simulink model "Disturbance_LQG_Stabilization_Simulink_Offline_Pendulum_Control"  (R2022b)
settings: Solver=VariableStepAuto  StartTime=0.0  StopTime=30  RelTol=1e-3
undefined symbols (not defined in the file or in its folder): A, A_kf, A_ob, B, B_kf, B_ob, C_full, C_kf, C_ob, D_full, D_kf, D_ob, K_lq, K_lq_alpha, Kpp, sigbuilder_block, voltage_max, x0
settings Model: Creator=utente  LastModifiedBy=federicocorso
settings SolverCC: AlgebraicLoopSolver=TrustRegion
settings DebuggingCC: UnconnectedInputMsg=warning  UnconnectedOutputMsg=warning  UnconnectedLineMsg=warning  SFMachineParentedDataDiag=warning
settings ModelReferenceCC: EnableRefExpFcnMdlSchedulingChecks=on

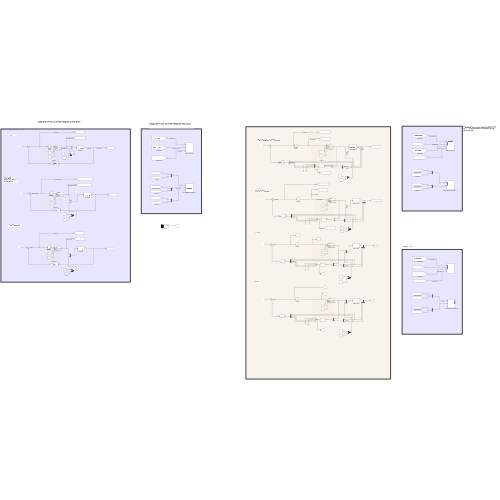
[thumbnail: Simulink's stored preview of the top-level diagram]
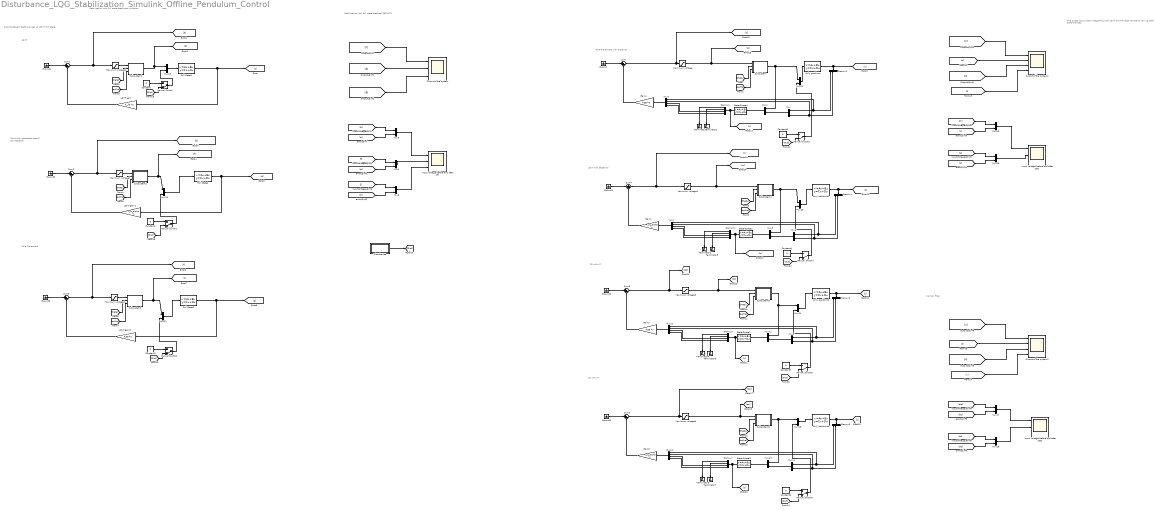
== system Disturbance_LQG_Stabilization_Simulink_Offline_Pendulum_Control ==
  note: LQ with KF
  note: PP with KF
  note: The closed loop system integrating both LQinf and PP observer seems having satisfactory performances.
  note: Kalman Filter
  note: Pole Placement with Observer
  note: Stabilization with full state feedback simulation
  note: LQinf
  note: Pole Placement Performances VS LQinf: Full State
  note: LQinf with prescribed rate of convergence
  note: Pole Placement
  note: Stabilization with full state feedback RESULTS
  note: LQinf with Observer
  Constant{,1..6} (7 alike) : Constant  Value=0
  Demux{1..8} (8 alike) : Demux
  Disturbance : Subsystem  Tag=STV Subsys  LoadFcn=sigbuilder_block('load',[516 294 550 400 ]);  StartFcn=sigbuilder_block('start');  StopFcn=sigbuilder_block('stop');  ClipboardFcn=sigbuilder_block('clipboard');  mask(Sigbuilder block){tuvar=[0:10]}
      mask help: Simulink:masks:SigbuilderBlock_MD
      mask init:
      | if ~strcmp(get_param(bdroot(gcbh),'SimulationStatus'),'stopped') tuvar = sigbuilder_block('maskInit'); end
      settings: CopyFcn=sigbuilder_block('copy');  DeleteFcn=sigbuilder_block('delete');  ModelCloseFcn=sigbuilder_block('modelClose');  PreSaveFcn=sigbuilder_block('preSave');  PauseFcn=sigbuilder_block('pause');  ContinueFcn=sigbuilder_block('continue');  NameChangeFcn=sigbuilder_block('namechange');  OpenFcn=sigbuilder_block('open',[516 294 550 400 ]);  CloseFcn=sigbuilder_block('close');
      mask Display: plot(0, 0, 100, 100,[2, 2, 32, 32, 2], [68, 8, 8, 68, 68],[32, 2], [38, 38], [32, 19, 2],[53, 60, 44], [32, 17, 17, 2],[16, 16, 31, 31]);txt = getActiveGroup(gcbh);text(2, 100, txt,'verticalAlignment', 'top');
  Full State1 : StateSpace  A=A  B=B  C=C_full  D=D_full  InitialCondition=x0
  Full State2 : StateSpace  A=A  B=B  C=C_full  D=D_full  InitialCondition=x0
  Full State3 : StateSpace  A=A  B=B  C=C_full  D=D_full  InitialCondition=x0
  Gain1 : Gain  Gain=K_lq_alpha  Multiplication=Matrix(K*u) (u vector)
  Gain2 : Gain  Gain=Kpp  Multiplication=Matrix(K*u) (u vector)
  Gain3 : Gain  Gain=K_lq_alpha  Multiplication=Matrix(K*u) (u vector)
  Gain4 : Gain  Gain=Kpp  Multiplication=Matrix(K*u) (u vector)
  Ground{,1..6} (7 alike) : Ground
  Input Voltage before and after sat : Scope  NumInputPorts=3
  Input Voltage before and after sat1 : Scope  NumInputPorts=3
  Input Voltage before and after sat2 : Scope  NumInputPorts=3
  LQinf gain : Gain  Gain=K_lq  Multiplication=Matrix(K*u) (u vector)
  LQinf gain1 : Gain  Gain=K_lq_alpha  Multiplication=Matrix(K*u) (u vector)
  LQinf gain2 : Gain  Gain=Kpp  Multiplication=Matrix(K*u) (u vector)
  Manual Switch{,1..6} (7 alike) : ManualSwitch  CurrentSetting=0
  Maximum voltage{,1..6} (7 alike) : Saturate  UpperLimit=voltage_max  LowerLimit=-voltage_max
  Mux{,2..6,8..9,11,13..25} (22 alike) : Mux  Inputs=2
  Mux{1,7,10,12} (4 alike) : Mux
  Only positions{,1..3} (4 alike) : StateSpace  A=A  B=B  C=C_full  D=D_full  InitialCondition=x0
  Output of the system : Scope  NumInputPorts=3
  Output of the system1 : Scope  NumInputPorts=4
  Output of the system2 : Scope  NumInputPorts=4
  State-Space1 : StateSpace  A=A_ob  B=B_ob  C=C_ob  D=D_ob  InitialCondition=[0;0;0;0]
  State-Space2 : StateSpace  A=A_kf  B=B_kf  C=C_kf  D=D_kf  InitialCondition=[0;0;0;0]
  State-Space3 : StateSpace  A=A_kf  B=B_kf  C=C_kf  D=D_kf  InitialCondition=[0;0;0;0]
  State-Space4 : StateSpace  A=A_ob  B=B_ob  C=C_ob  D=D_ob  InitialCondition=[0;0;0;0]
  Subsystem : Subsystem
  Subsystem1 : Subsystem
  Subsystem2 : Subsystem
  Subsystem3 : Subsystem
  Subsystem4 : Subsystem
  Subsystem5 : Subsystem
  Subsystem6 : Subsystem
  Sum{,1..6} (7 alike) : Sum  Inputs=|+-
  Terminator{,1..7} (8 alike) : Terminator
  wires:
  Maximum voltage/1 -> Subsystem/1(Control), [p]  "input Voltage PP"
  [theta] -> Subsystem/2(Theta)
  [aplha] -> Subsystem/3(Alpha)
  Ground/1 -> Sum/1
  Sum/1 -> [o], Maximum voltage/1  "erroro PP"
  Gain4/1 -> Sum/2
  Mux2/1 -> State-Space4/1  "Estimated States"
  State-Space4/1 -> [r], Demux1/1  "PP est"
  Subsystem/1(control) -> Mux2/1, Mux22/1
  Sum1/1 -> Maximum voltage1/1, [a]  "error LQinf"
  Ground1/1 -> Sum1/1
  Full State1/1 -> [c], LQinf gain/1  "Output LQinf"
  Subsystem1/1(control) -> [b], Mux19/1  "Input Voltage LQinf"
  Maximum voltage1/1 -> Subsystem1/1(Control)
  [aplha] -> Subsystem1/3(Alpha)
  [theta] -> Subsystem1/2(Theta)
  LQinf gain/1 -> Sum1/2
  Only positions/1 -> [n], Demux2/1  "Output PP"
  Mux/1 -> Mux2/2
  Demux2/2 -> Mux/2, Mux1/2  "alpha_sim"
  Demux2/1 -> Mux/1, Mux1/1  "theta_sim"
  Mux1/1 -> Gain4/1
  Demux1/3 -> Mux1/3
  Demux1/4 -> Mux1/4
  Demux1/1 -> Terminator/1
  Demux1/2 -> Terminator1/1
  [c] -> Output of the system/1  "Output LQinf"
  [b] -> Mux3/1
  [a] -> Mux3/2
  Mux3/1 -> Input Voltage before and after sat/1  "LQinf"
  Ground2/1 -> Sum2/1
  Full State2/1 -> [d], LQinf gain1/1  "Output LQinf_alpha"
  Sum2/1 -> Maximum voltage2/1, [e]  "error LQinf_alpha"
  Maximum voltage2/1 -> Subsystem2/1(Control)
  [aplha] -> Subsystem2/3(Alpha)
  LQinf gain1/1 -> Sum2/2
  Subsystem2/1(control) -> [f], Mux20/1  "Input Voltage LQinf_alpha"
  [theta] -> Subsystem2/2(Theta)
  [theta] -> Subsystem3/2(Theta)
  LQinf gain2/1 -> Sum3/2
  Sum3/1 -> Maximum voltage3/1, [h]  "error PP"
  Full State3/1 -> [g], LQinf gain2/1  "Output PP"
  Maximum voltage3/1 -> Subsystem3/1(Control)
  [aplha] -> Subsystem3/3(Alpha)
  Ground3/1 -> Sum3/1
  Subsystem3/1(control) -> [j], Mux21/1  "Input Voltage PP"
  [e] -> Mux4/2
  [f] -> Mux4/1
  Mux4/1 -> Input Voltage before and after sat/2  "LQinf_alpha"
  Mux5/1 -> Input Voltage before and after sat/3  "PP"
  [j] -> Mux5/1
  [h] -> Mux5/2
  [d] -> Output of the system/2  "Output LQinf_alpha"
  [g] -> Output of the system/3  "Output PP"
  Demux3/2 -> Terminator3/1
  Demux3/1 -> Terminator2/1
  Demux3/4 -> Mux7/4
  Demux3/3 -> Mux7/3
  Mux7/1 -> Gain1/1
  Demux4/1 -> Mux7/1, Mux6/1  "theta_sim"
  Demux4/2 -> Mux7/2, Mux6/2  "alpha_sim"
  Mux6/1 -> Mux8/2
  Only positions1/1 -> [k], Demux4/1  "Output LQinf"
  Subsystem4/1(control) -> Mux23/1, Mux8/1
  State-Space1/1 -> [q], Demux3/1  "LQinf est"
  Mux8/1 -> State-Space1/1  "Estimated States"
  Gain1/1 -> Sum4/2
  Sum4/1 -> Maximum voltage4/1, [l]  "error LQinf"
  Ground4/1 -> Sum4/1
  [aplha] -> Subsystem4/3(Alpha)
  [theta] -> Subsystem4/2(Theta)
  Maximum voltage4/1 -> Subsystem4/1(Control), [m]  "input Voltage LQinf"
  Maximum voltage5/1 -> [cc], Subsystem5/1(Control)
  [theta] -> Subsystem5/2(Theta)
  [aplha] -> Subsystem5/3(Alpha)
  Ground5/1 -> Sum5/1
  Sum5/1 -> [dd], Maximum voltage5/1  "not sat"
  Gain2/1 -> Sum5/2
  Mux11/1 -> State-Space2/1  "Estimated States"
  State-Space2/1 -> [v], Demux5/1
  Subsystem5/1(control) -> Mux24/1, Mux11/1
  Only positions2/1 -> [u], Demux6/1
  Mux9/1 -> Mux11/2
  Demux6/2 -> Mux9/2, Mux10/2  "alpha_sim"
  Demux6/1 -> Mux9/1, Mux10/1  "theta_sim"
  Mux10/1 -> Gain2/1
  Demux5/3 -> Mux10/3
  Demux5/4 -> Mux10/4
  Demux5/1 -> Terminator4/1
  Demux5/2 -> Terminator5/1
  Demux7/2 -> Terminator7/1
  Demux7/1 -> Terminator6/1
  Demux7/4 -> Mux12/4
  Demux7/3 -> Mux12/3
  Mux12/1 -> Gain3/1
  Demux8/1 -> Mux12/1, Mux14/1  "theta_sim"
  Demux8/2 -> Mux12/2, Mux14/2  "alpha_sim"
  Mux14/1 -> Mux13/2
  Only positions3/1 -> [s], Demux8/1
  Subsystem6/1(control) -> Mux25/1, Mux13/1
  State-Space3/1 -> [t], Demux7/1
  Mux13/1 -> State-Space3/1  "Estimated States"
  Gain3/1 -> Sum6/2
  Sum6/1 -> [bb], Maximum voltage6/1  "not sat"
  Ground6/1 -> Sum6/1
  [aplha] -> Subsystem6/3(Alpha)
  [theta] -> Subsystem6/2(Theta)
  Maximum voltage6/1 -> [aa], Subsystem6/1(Control)
  [n] -> Output of the system1/3  "Output PP sim"
  Mux16/1 -> Input Voltage before and after sat1/2  "PP"
  [p] -> Mux16/1
  [o] -> Mux16/2
  Mux15/1 -> Input Voltage before and after sat1/1  "LQinf"
  [l] -> Mux15/2
  [m] -> Mux15/1
  [k] -> Output of the system1/1  "Output LQinf sim"
  [q] -> Output of the system1/2  "Output LQinf est"
  [r] -> Output of the system1/4  "Output PP est"
  [v] -> Output of the system2/4  "Output PP est"
  [t] -> Output of the system2/2  "Output LQinf est"
  [s] -> Output of the system2/1  "Output LQinf sim"
  [aa] -> Mux17/1
  [bb] -> Mux17/2
  Mux17/1 -> Input Voltage before and after sat2/1  "LQinf"
  [dd] -> Mux18/2
  [cc] -> Mux18/1
  Mux18/1 -> Input Voltage before and after sat2/2  "PP"
  [u] -> Output of the system2/3  "Output PP sim"
  Mux19/1 -> Full State1/1
  Manual Switch/1 -> Mux19/2
  Manual Switch1/1 -> Mux20/2
  Manual Switch2/1 -> Mux21/2
  Manual Switch3/1 -> Mux22/2
  Manual Switch4/1 -> Mux23/2
  Manual Switch5/1 -> Mux24/2
  Mux24/1 -> Only positions2/1
  Mux23/1 -> Only positions1/1
  Mux22/1 -> Only positions/1
  Manual Switch6/1 -> Mux25/2
  Mux25/1 -> Only positions3/1
  Mux21/1 -> Full State3/1
  Mux20/1 -> Full State2/1
  [Dist] -> Manual Switch/2
  Constant/1 -> Manual Switch/1
  Constant2/1 -> Manual Switch2/1
  [Dist] -> Manual Switch2/2
  Constant1/1 -> Manual Switch1/1
  Constant3/1 -> Manual Switch3/1
  [Dist] -> Manual Switch3/2
  [Dist] -> Manual Switch4/2
  Constant4/1 -> Manual Switch4/1
  Constant5/1 -> Manual Switch5/1
  [Dist] -> Manual Switch5/2
  [Dist] -> Manual Switch6/2
  Constant6/1 -> Manual Switch6/1
  Disturbance/1(Signal 2) -> [Dist]
  [Dist] -> Manual Switch1/2

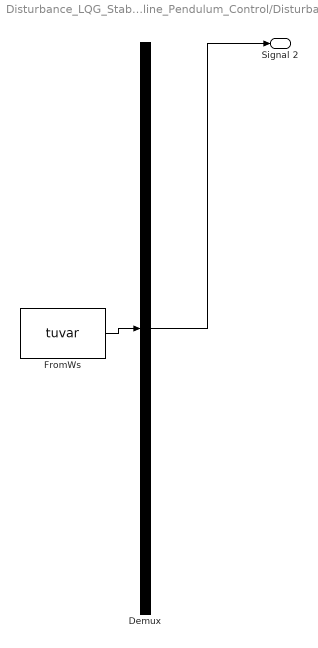
== system Disturbance_LQG_Stabilization_Simulink_Offline_Pendulum_Control/Disturbance ==
  Demux : Demux  Tag=STV Demux  Outputs=1
      settings: DisplayOption=none
  FromWs : FromWorkspace  Tag=STV FromWs  VariableName=tuvar
      SigBuilderData=|
      | common.afterFinalStr = 'Extrapolate'
      | common.sampleTime = 0
      | dataSet.timeRange = [0 10]
      | dataSet.name = 'Group 1'
      | sbobj.Groups.Name = 'Group 1'
      | sbobj.Groups.Signals.Name = 'Signal 2'
      | sbobj.Groups.Signals.XData = [0 4 4 4.01 4.01 10]
      | sbobj.Groups.Signals.YData = [0 0 0.2 0.2 0 0]
  Signal 2 : Outport  Tag=STV Outport
  wires:
  Demux/1 -> Signal 2/1
  FromWs/1 -> Demux/1

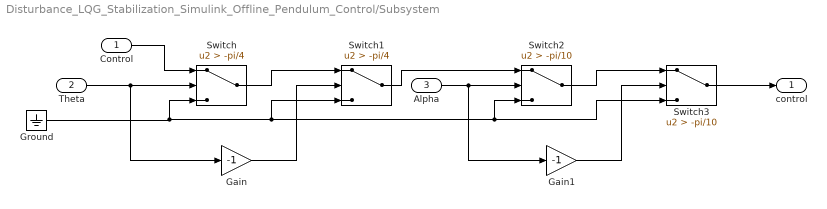
== system Disturbance_LQG_Stabilization_Simulink_Offline_Pendulum_Control/Subsystem ==
  Control : Inport
  Theta : Inport  Port=2
  Alpha : Inport  Port=3
  Gain : Gain  Gain=-1
  Gain1 : Gain  Gain=-1
  Ground : Ground
  Switch : Switch  Criteria=u2 > Threshold  Threshold=-pi/4  SaturateOnIntegerOverflow=off  InputSameDT=off
  Switch1 : Switch  Criteria=u2 > Threshold  Threshold=-pi/4  SaturateOnIntegerOverflow=off  InputSameDT=off
  Switch2 : Switch  Criteria=u2 > Threshold  Threshold=-pi/10  SaturateOnIntegerOverflow=off  InputSameDT=off
  Switch3 : Switch  Criteria=u2 > Threshold  Threshold=-pi/10  SaturateOnIntegerOverflow=off  InputSameDT=off
  control : Outport
  wires:
  Gain/1 -> Switch1/2
  Theta/1 -> Gain/1, Switch/2
  Control/1 -> Switch/1
  Switch/1 -> Switch1/1
  Gain1/1 -> Switch3/2
  Switch1/1 -> Switch2/1
  Ground/1 -> Switch3/3, Switch2/3, Switch1/3, Switch/3
  Switch2/1 -> Switch3/1
  Alpha/1 -> Switch2/2, Gain1/1
  Switch3/1 -> control/1

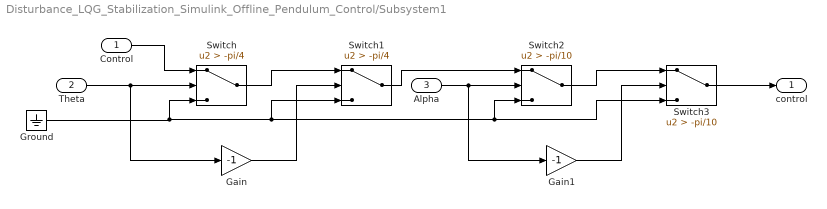
== system Disturbance_LQG_Stabilization_Simulink_Offline_Pendulum_Control/Subsystem1 ==
  Control : Inport
  Theta : Inport  Port=2
  Alpha : Inport  Port=3
  Gain : Gain  Gain=-1
  Gain1 : Gain  Gain=-1
  Ground : Ground
  Switch : Switch  Criteria=u2 > Threshold  Threshold=-pi/4  SaturateOnIntegerOverflow=off  InputSameDT=off
  Switch1 : Switch  Criteria=u2 > Threshold  Threshold=-pi/4  SaturateOnIntegerOverflow=off  InputSameDT=off
  Switch2 : Switch  Criteria=u2 > Threshold  Threshold=-pi/10  SaturateOnIntegerOverflow=off  InputSameDT=off
  Switch3 : Switch  Criteria=u2 > Threshold  Threshold=-pi/10  SaturateOnIntegerOverflow=off  InputSameDT=off
  control : Outport
  wires:
  Gain/1 -> Switch1/2
  Theta/1 -> Gain/1, Switch/2
  Control/1 -> Switch/1
  Switch/1 -> Switch1/1
  Gain1/1 -> Switch3/2
  Switch1/1 -> Switch2/1
  Ground/1 -> Switch3/3, Switch2/3, Switch1/3, Switch/3
  Switch2/1 -> Switch3/1
  Alpha/1 -> Switch2/2, Gain1/1
  Switch3/1 -> control/1

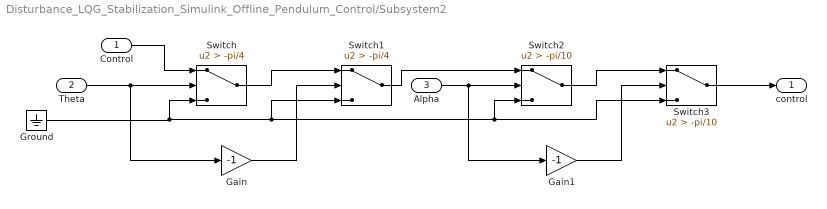
== system Disturbance_LQG_Stabilization_Simulink_Offline_Pendulum_Control/Subsystem2 ==
  Control : Inport
  Theta : Inport  Port=2
  Alpha : Inport  Port=3
  Gain : Gain  Gain=-1
  Gain1 : Gain  Gain=-1
  Ground : Ground
  Switch : Switch  Criteria=u2 > Threshold  Threshold=-pi/4  SaturateOnIntegerOverflow=off  InputSameDT=off
  Switch1 : Switch  Criteria=u2 > Threshold  Threshold=-pi/4  SaturateOnIntegerOverflow=off  InputSameDT=off
  Switch2 : Switch  Criteria=u2 > Threshold  Threshold=-pi/10  SaturateOnIntegerOverflow=off  InputSameDT=off
  Switch3 : Switch  Criteria=u2 > Threshold  Threshold=-pi/10  SaturateOnIntegerOverflow=off  InputSameDT=off
  control : Outport
  wires:
  Gain/1 -> Switch1/2
  Theta/1 -> Gain/1, Switch/2
  Control/1 -> Switch/1
  Switch/1 -> Switch1/1
  Gain1/1 -> Switch3/2
  Switch1/1 -> Switch2/1
  Ground/1 -> Switch3/3, Switch2/3, Switch1/3, Switch/3
  Switch2/1 -> Switch3/1
  Alpha/1 -> Switch2/2, Gain1/1
  Switch3/1 -> control/1

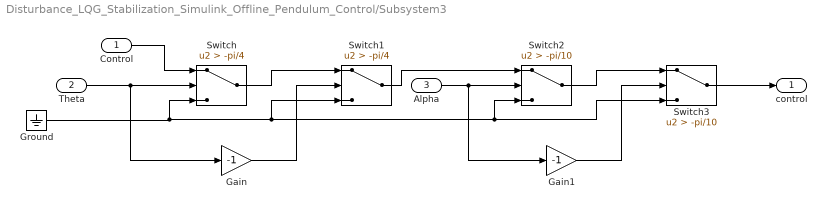
== system Disturbance_LQG_Stabilization_Simulink_Offline_Pendulum_Control/Subsystem3 ==
  Control : Inport
  Theta : Inport  Port=2
  Alpha : Inport  Port=3
  Gain : Gain  Gain=-1
  Gain1 : Gain  Gain=-1
  Ground : Ground
  Switch : Switch  Criteria=u2 > Threshold  Threshold=-pi/4  SaturateOnIntegerOverflow=off  InputSameDT=off
  Switch1 : Switch  Criteria=u2 > Threshold  Threshold=-pi/4  SaturateOnIntegerOverflow=off  InputSameDT=off
  Switch2 : Switch  Criteria=u2 > Threshold  Threshold=-pi/10  SaturateOnIntegerOverflow=off  InputSameDT=off
  Switch3 : Switch  Criteria=u2 > Threshold  Threshold=-pi/10  SaturateOnIntegerOverflow=off  InputSameDT=off
  control : Outport
  wires:
  Gain/1 -> Switch1/2
  Theta/1 -> Gain/1, Switch/2
  Control/1 -> Switch/1
  Switch/1 -> Switch1/1
  Gain1/1 -> Switch3/2
  Switch1/1 -> Switch2/1
  Ground/1 -> Switch3/3, Switch2/3, Switch1/3, Switch/3
  Switch2/1 -> Switch3/1
  Alpha/1 -> Switch2/2, Gain1/1
  Switch3/1 -> control/1

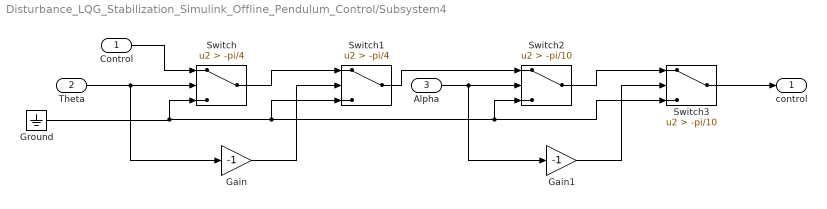
== system Disturbance_LQG_Stabilization_Simulink_Offline_Pendulum_Control/Subsystem4 ==
  Control : Inport
  Theta : Inport  Port=2
  Alpha : Inport  Port=3
  Gain : Gain  Gain=-1
  Gain1 : Gain  Gain=-1
  Ground : Ground
  Switch : Switch  Criteria=u2 > Threshold  Threshold=-pi/4  SaturateOnIntegerOverflow=off  InputSameDT=off
  Switch1 : Switch  Criteria=u2 > Threshold  Threshold=-pi/4  SaturateOnIntegerOverflow=off  InputSameDT=off
  Switch2 : Switch  Criteria=u2 > Threshold  Threshold=-pi/10  SaturateOnIntegerOverflow=off  InputSameDT=off
  Switch3 : Switch  Criteria=u2 > Threshold  Threshold=-pi/10  SaturateOnIntegerOverflow=off  InputSameDT=off
  control : Outport
  wires:
  Switch3/1 -> control/1
  Alpha/1 -> Gain1/1, Switch2/2
  Switch2/1 -> Switch3/1
  Ground/1 -> Switch/3, Switch1/3, Switch2/3, Switch3/3
  Switch1/1 -> Switch2/1
  Gain1/1 -> Switch3/2
  Switch/1 -> Switch1/1
  Control/1 -> Switch/1
  Theta/1 -> Switch/2, Gain/1
  Gain/1 -> Switch1/2

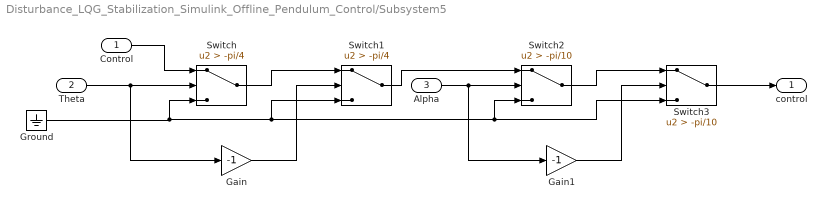
== system Disturbance_LQG_Stabilization_Simulink_Offline_Pendulum_Control/Subsystem5 ==
  Control : Inport
  Theta : Inport  Port=2
  Alpha : Inport  Port=3
  Gain : Gain  Gain=-1
  Gain1 : Gain  Gain=-1
  Ground : Ground
  Switch : Switch  Criteria=u2 > Threshold  Threshold=-pi/4  SaturateOnIntegerOverflow=off  InputSameDT=off
  Switch1 : Switch  Criteria=u2 > Threshold  Threshold=-pi/4  SaturateOnIntegerOverflow=off  InputSameDT=off
  Switch2 : Switch  Criteria=u2 > Threshold  Threshold=-pi/10  SaturateOnIntegerOverflow=off  InputSameDT=off
  Switch3 : Switch  Criteria=u2 > Threshold  Threshold=-pi/10  SaturateOnIntegerOverflow=off  InputSameDT=off
  control : Outport
  wires:
  Gain/1 -> Switch1/2
  Theta/1 -> Gain/1, Switch/2
  Control/1 -> Switch/1
  Switch/1 -> Switch1/1
  Gain1/1 -> Switch3/2
  Switch1/1 -> Switch2/1
  Ground/1 -> Switch3/3, Switch2/3, Switch1/3, Switch/3
  Switch2/1 -> Switch3/1
  Alpha/1 -> Switch2/2, Gain1/1
  Switch3/1 -> control/1

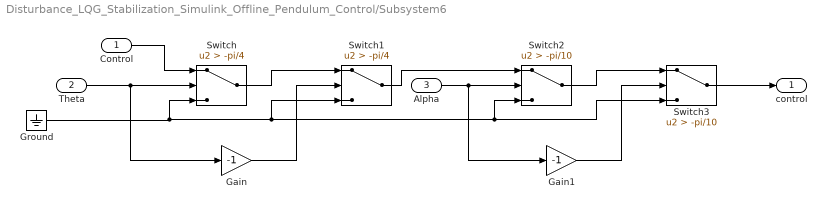
== system Disturbance_LQG_Stabilization_Simulink_Offline_Pendulum_Control/Subsystem6 ==
  Control : Inport
  Theta : Inport  Port=2
  Alpha : Inport  Port=3
  Gain : Gain  Gain=-1
  Gain1 : Gain  Gain=-1
  Ground : Ground
  Switch : Switch  Criteria=u2 > Threshold  Threshold=-pi/4  SaturateOnIntegerOverflow=off  InputSameDT=off
  Switch1 : Switch  Criteria=u2 > Threshold  Threshold=-pi/4  SaturateOnIntegerOverflow=off  InputSameDT=off
  Switch2 : Switch  Criteria=u2 > Threshold  Threshold=-pi/10  SaturateOnIntegerOverflow=off  InputSameDT=off
  Switch3 : Switch  Criteria=u2 > Threshold  Threshold=-pi/10  SaturateOnIntegerOverflow=off  InputSameDT=off
  control : Outport
  wires:
  Switch3/1 -> control/1
  Alpha/1 -> Gain1/1, Switch2/2
  Switch2/1 -> Switch3/1
  Ground/1 -> Switch/3, Switch1/3, Switch2/3, Switch3/3
  Switch1/1 -> Switch2/1
  Gain1/1 -> Switch3/2
  Switch/1 -> Switch1/1
  Control/1 -> Switch/1
  Theta/1 -> Switch/2, Gain/1
  Gain/1 -> Switch1/2
